simulink model "OptimalSlidingMode"  (Simulink 7.4)
settings: Solver=ode5  StartTime=0.0  StopTime=2  FixedStep=.001  MaxStep=.001  MinStep=.001  RelTol=1e-3
libraries: simulink x2
settings Model: Creator=Home  LastModifiedBy=Jupiter  SimulationMode=accelerator
settings OptimizationCC: InitFltsAndDblsToZero=on

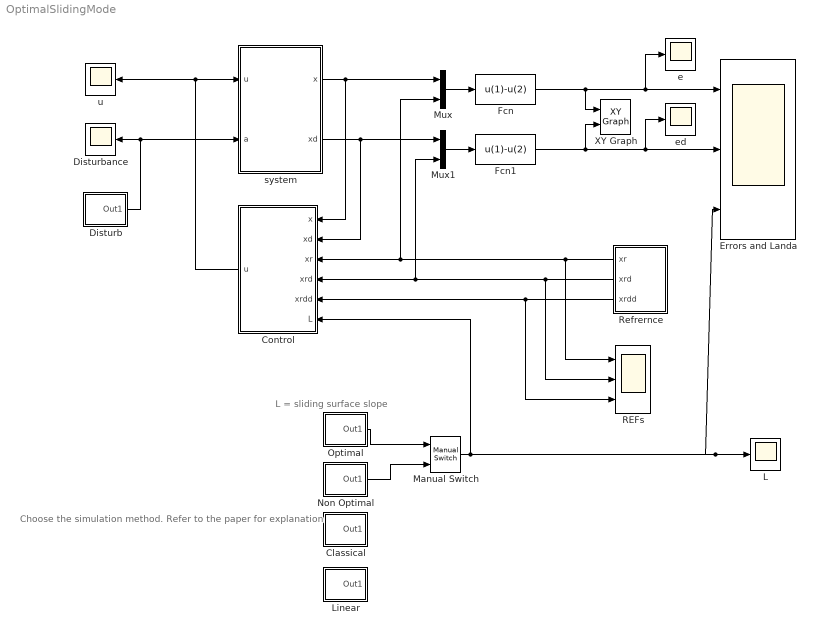
== system OptimalSlidingMode ==
  note: L = sliding surface slope
  note: Choose the simulation method.
      | Refer to the paper for explanation
  Classical : Subsystem
  Control : Subsystem
  Disturb : Subsystem
  Disturbance : Scope
      settings: SaveName=ScopeData2
  Errors and Landa : Scope  NumInputPorts=3
      settings: TimeRange=2  YMin=-5e-005~-0.002~2  YMax=0.00035~0.00075~20  SaveName=er  DataFormat=Structure
  Fcn : Fcn  Expr=u(1)-u(2)
  Fcn1 : Fcn  Expr=u(1)-u(2)
  L : Scope
      settings: YMin=2  YMax=20  SaveName=L  DataFormat=Structure
  Linear : Subsystem
  Manual Switch : simulink/Signal Routing/Manual Switch  SystemSampleTime=-1  sw=0  action=0  varsize=off
  Mux : Mux  Inputs=2
  Mux1 : Mux  Inputs=2
  "Non Optimal " : Subsystem
  Optimal : Subsystem
  REFs : Scope  NumInputPorts=3
      settings: YMin=-5~-5~-5  YMax=5~5~5  SaveName=ScopeData3
  Refrernce : Subsystem
  XY Graph : simulink/Sinks/XY Graph  SystemSampleTime=-1  xmin=-.0005  xmax=.0005  ymin=-.005  ymax=.005  st=-1
  e : Scope
      settings: YMin=-5e-005  YMax=0.0003  SaveName=e  DataFormat=Structure
  ed : Scope
      settings: YMin=-0.0045  YMax=0.0005  SaveName=ed  DataFormat=Structure
  system : Subsystem
  u : Scope
      settings: YMin=0.5  YMax=4.75  SaveName=U  DataFormat=Structure
  wires:
  system/1(x) -> Mux/1, Control/1(x)
  Disturb/1(Out1) -> system/2(a), Disturbance/1
  system/2(xd) -> Control/2(xd), Mux1/1
  Refrernce/1(xr) -> REFs/1, Control/3(xr), Mux/2
  Refrernce/2(xrd) -> REFs/2, Control/4(xrd), Mux1/2
  Refrernce/3(xrdd) -> Control/5(xrdd), REFs/3
  Mux/1 -> Fcn/1
  Fcn/1 -> XY Graph/1, e/1, Errors and Landa/1
  Mux1/1 -> Fcn1/1
  Fcn1/1 -> ed/1, Errors and Landa/2, XY Graph/2
  Control/1(u) -> system/1(u), u/1
  Optimal/1(Out1) -> Manual Switch/1
  Manual Switch/1 -> Control/6(L), L/1, Errors and Landa/3
  "Non Optimal "/1(Out1) -> Manual Switch/2

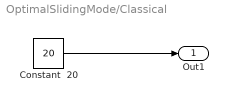
== system OptimalSlidingMode/Classical ==
  Constant  20 : Constant  Value=20  OutDataType=sfix(16)  OutScaling=2^0
  Out1 : Outport
  wires:
  Constant  20/1 -> Out1/1

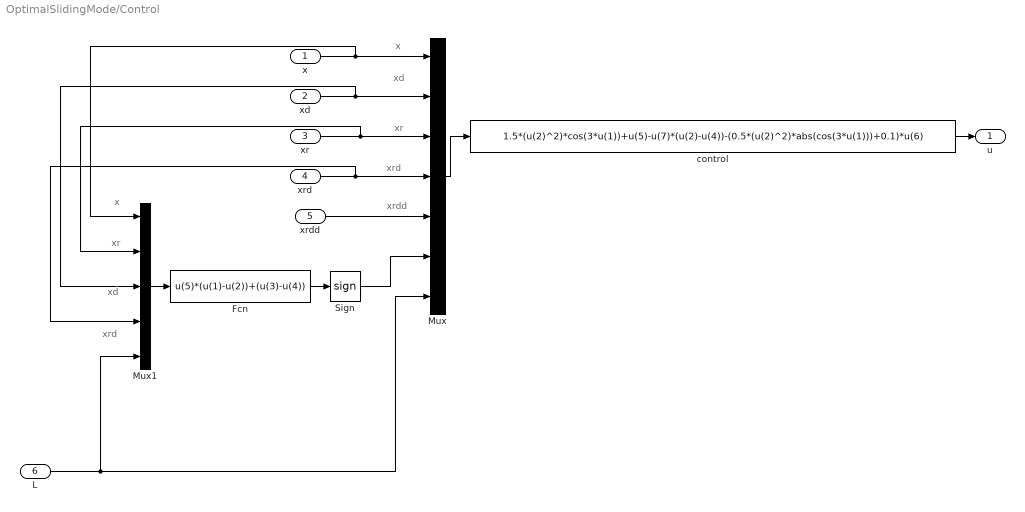
== system OptimalSlidingMode/Control ==
  note: xd
  note: x
  note: xr
  note: xd
  note: xrd
  note: xrdd
  note: xrd
  note: xr
  note: x
  x : Inport
  xd : Inport  Port=2
  xr : Inport  Port=3
  xrd : Inport  Port=4
  xrdd : Inport  Port=5
  L : Inport  Port=6
  Fcn : Fcn  Expr=u(5)*(u(1)-u(2))+(u(3)-u(4))
  Mux : Mux  Inputs=7
  Mux1 : Mux  Inputs=5
  Sign : Signum
  control : Fcn  Expr=1.5*(u(2)^2)*cos(3*u(1))+u(5)-u(7)*(u(2)-u(4))-(0.5*(u(2)^2)*abs(cos(3*u(1)))+0.1)*u(6)
  u : Outport
  wires:
  Mux/1 -> control/1
  x/1 -> Mux/1, Mux1/1
  xd/1 -> Mux/2, Mux1/3
  xr/1 -> Mux/3, Mux1/2
  control/1 -> u/1
  xrd/1 -> Mux/4, Mux1/4
  xrdd/1 -> Mux/5
  Mux1/1 -> Fcn/1
  Fcn/1 -> Sign/1
  Sign/1 -> Mux/6
  L/1 -> Mux/7, Mux1/5

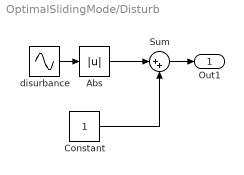
== system OptimalSlidingMode/Disturb ==
  Abs : Abs  OutDataType=sfix(16)  OutScaling=2^0
  Constant : Constant  OutDataType=sfix(16)  OutScaling=2^0
  Sum : Sum  Inputs=|++  OutDataType=sfix(16)  OutScaling=2^0
  disurbance : Sin  Amplitude=1  Bias=0  Frequency=1  Phase=0  Samples=10  SampleTime=0  Offset=0
  Out1 : Outport
  wires:
  Constant/1 -> Sum/2
  disurbance/1 -> Abs/1
  Abs/1 -> Sum/1
  Sum/1 -> Out1/1

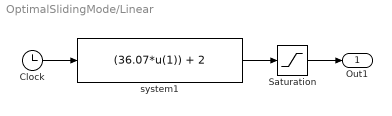
== system OptimalSlidingMode/Linear ==
  Clock : Clock
      settings: Decimation=10
  Saturation : Saturate  UpperLimit=20  OutDataType=sfix(16)  OutScaling=2^0
  system1 : Fcn  Expr=(36.07*u(1)) + 2
  Out1 : Outport
  wires:
  Clock/1 -> system1/1
  system1/1 -> Saturation/1
  Saturation/1 -> Out1/1

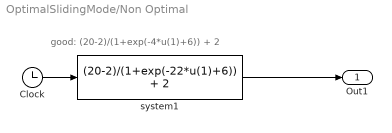
== system OptimalSlidingMode/Non Optimal  ==
  note: good: (20-2)/(1+exp(-4*u(1)+6)) + 2
  Clock : Clock
      settings: Decimation=10
  system1 : Fcn  Expr=(20-2)/(1+exp(-22*u(1)+6)) + 2
  Out1 : Outport
  wires:
  Clock/1 -> system1/1
  system1/1 -> Out1/1

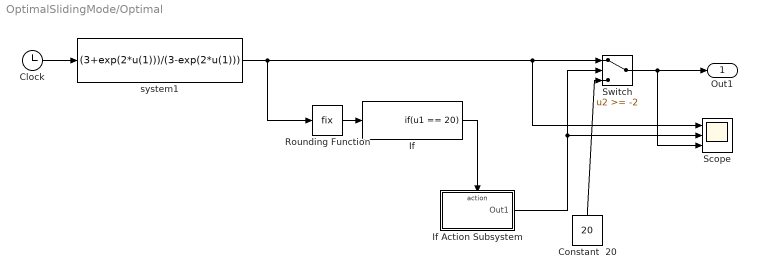
== system OptimalSlidingMode/Optimal ==
  Clock : Clock
      settings: Decimation=10
  Constant  20 : Constant  Value=20  OutDataType=sfix(16)  OutScaling=2^0
  If : If  IfExpression=u1 == 20  ShowElse=off
  If Action Subsystem : Subsystem  TreatAsAtomicUnit=on
  Rounding Function : Rounding  Operator=fix
  Scope : Scope  NumInputPorts=3
      settings: YMin=-1~0~-5  YMax=1~17.5~5  SaveName=S1
  Switch : Switch  Threshold=-2  OutDataType=sfix(16)  OutScaling=2^0
  system1 : Fcn  Expr=(3+exp(2*u(1)))/(3-exp(2*u(1)))
  Out1 : Outport
  wires:
  Switch/1 -> Out1/1, Scope/3
  Clock/1 -> system1/1
  system1/1 -> Rounding Function/1, Switch/1, Scope/1
  If Action Subsystem/1(Out1) -> Switch/2, Scope/2
  Constant  20/1 -> Switch/3
  Rounding Function/1 -> If/1
  If/1 -> If Action Subsystem/Action

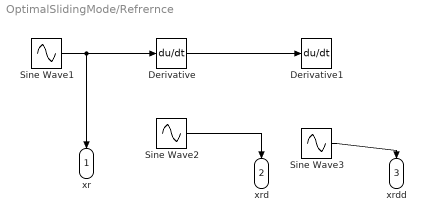
== system OptimalSlidingMode/Refrernce ==
  Derivative : Derivative
  Derivative1 : Derivative
  Sine Wave1 : Sin  Amplitude=1  Bias=0  Frequency=pi/2  Phase=0  Samples=10  SampleTime=0  Offset=0
  Sine Wave2 : Sin  Amplitude=pi/2  Bias=0  Frequency=pi/2  Phase=pi/2  Samples=10  SampleTime=0  Offset=0
  Sine Wave3 : Sin  Amplitude=-(pi/2)*(pi/2)  Bias=0  Frequency=pi/2  Phase=0  Samples=10  SampleTime=0  Offset=0
  xr : Outport
  xrd : Outport  Port=2
  xrdd : Outport  Port=3
  wires:
  Sine Wave1/1 -> xr/1, Derivative/1
  Derivative/1 -> Derivative1/1
  Sine Wave3/1 -> xrdd/1
  Sine Wave2/1 -> xrd/1

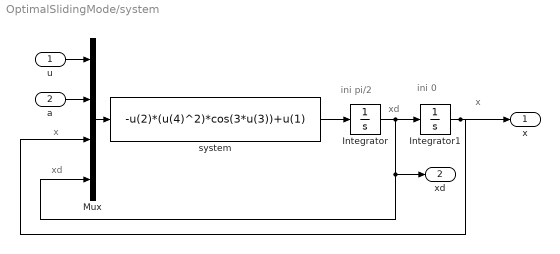
== system OptimalSlidingMode/system ==
  note: xd
  note: x
  note: xd
  note: x
  note: ini 0
  note: ini pi/2
  u : Inport
  a : Inport  Port=2
  Integrator : Integrator  InitialCondition=pi/2 - 0.0006
  Integrator1 : Integrator  InitialCondition=.0003
  Mux : Mux
  system : Fcn  Expr=-u(2)*(u(4)^2)*cos(3*u(3))+u(1)
  x : Outport
  xd : Outport  Port=2
  wires:
  Mux/1 -> system/1
  u/1 -> Mux/1
  a/1 -> Mux/2
  system/1 -> Integrator/1
  Integrator/1 -> Integrator1/1, xd/1, Mux/4
  Integrator1/1 -> x/1, Mux/3

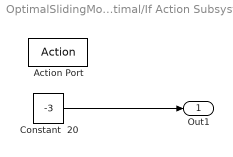
== system OptimalSlidingMode/Optimal/If Action Subsystem ==
  Action Port : ActionPort  ActionType=then
  Constant  20 : Constant  Value=-3  OutDataType=sfix(16)  OutScaling=2^0
  Out1 : Outport  OutDataType=sfix(16)  OutScaling=2^0
  wires:
  Constant  20/1 -> Out1/1
